simulink model "bball_2"  (R2021a)
settings: Solver=ode15s  StartTime=0.0  StopTime=timeFinal  MaxStep=timeStepMax  RelTol=1e-3
undefined symbols (not defined in the file): a1, a2
settings Model: Creator=amit  LastModifiedBy=amit

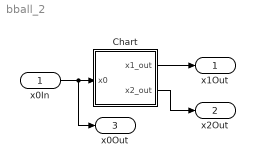
== system bball_2 ==
  x0In : Inport
  Chart : Stateflow chart  TreatAsAtomicUnit=on
  x1Out : Outport  SignalName=x1Out
  x2Out : Outport  Port=2  SignalName=x2Out
  x0Out : Outport  Port=3  SignalName=x0Out
  wires:
  x0In/1 -> Chart/1(x0), x0Out/1
  Chart/2(x2_out) -> x2Out/1
  Chart/1(x1_out) -> x1Out/1

== stateflow chart bball_2/Chart ==
  settings: updateMethod=CONTINUOUS  executeAtInitialization=1
  state loc1
    du:
    x1_dot = 0.0000000 * x0 + -0.0000000 * x1 + 1.0000000 * x2 + 0.0000000 * 1;
    x2_dot = 1.0000000 * x0 + 0.0000000 * x1 + 0.0000000 * x2 + 0.0000000 * 1;
    exit:
    x1_out = x1;
    x2_out = x2;
  (junction 2) -> loc1 : [1.0 * x0 + 17.770932524494636 * x1 + 0.009194766167857395 * x2 + 9.47353031898127 * 1 <= 0.000000 + 0]{x1 = 0.0000000 * x0 + 1.0000000 * x1 + 0.0000000 * x2 + 0.000; x2 = 0.0093004 * x0 + 0.4025997 * x1 + -0.7997943 * x2 + 0.036; }
  (default) -> loc1 : {x1 = a1; x2 = a2; }
  loc1 -> (junction 5) [order 2]
  (junction 5) -> loc1 : {x1 = x1; x2 = x2; }
  loc1 -> (junction 2) [order 1]
  data: x0 input; x1_out output; x2_out output; x1 local double; x2 local double; a1 parameter; a2 parameter
  data x1 settings: updateMethod=SF_CONTINUOUS_TIME_DATA
  data x2 settings: updateMethod=SF_CONTINUOUS_TIME_DATA
